simulink model "Lin_test_dsim_quant"  (R2012b)
settings: Solver=FixedStepDiscrete  SolverMode=SingleTasking  StartTime=0.0  StopTime=4096*15  RelTol=1e-3
undefined symbols (not defined in the file or in its folder): fft_stages
libraries: xbsIndex_r4 x7736, casper_library_misc x13, casper_library_sources x12, xps_library x1
(part 33 of 60)

== system Lin_test_dsim_quant/wng0/bus_mult ==
  a : Inport
  b : Inport  Port=2
  a*b_bussify : Subsystem  AncestorBlock=casper_library_flow_control/bus_create  mask(bus_create){inputNum=8}
      mask prompts: inputNum "Number of inputs:"
      mask init:
      | bus_create_init(gcb,...
      |     'inputNum', inputNum);
  a_debus : Subsystem  AncestorBlock=casper_library_flow_control/bus_expand  mask(bus_expand){mode=divisions of arbitrary size, outputNum=1, outputWidth=[21 21 21 21 21 21 21 21], outputBinaryPt=[18 18 18 18 18 18 18 18], outputArithmeticType=[1 1 1 1 1 1 1 1], show_format=on, outputToWorkspace=off, variablePrefix=, outputToModelAsWell=on}
      mask prompts: outputNum "Number of outputs:"; outputWidth "Output width [msb ... lsb]:"; outputBinaryPt "Output binary point position [msb ... lsb]:"; outputArithmeticType "Output arithmetic type (ufix=0, fix=1, bool=2) [msb ... lsb]:"; show_format "Print format string?"; outputToWorkspace "Output to workspace?"; variablePrefix "Variable name prefix:"; outputToModelAsWell "Output to model as well?"
      mask help:
      | Expands a 'bus' made using a bus_create or Xilinx
      | concat block.
      | The input will be divided into the specified number
      | of outputs with the specified arithmetic types.
      | Divisions are made from most significant bit.
      mask init: same as Lin_test_dsim_quant/bus_expand1
      settings: AttributesFormatString=8 outputs: f21.18,f21.18,f21.18,f21.18,f21.18,f21.18,f21.18,f21.18,
      mask TypeOptions mode: divisions of equal size | divisions of arbitrary size
      mask Callback mode: bus_expand_callback();
      mask Callback outputWidth: bus_expand_callback();
      mask Callback outputToWorkspace: bus_expand_callback();
  b_debus : Subsystem  AncestorBlock=casper_library_flow_control/bus_expand  mask(bus_expand){mode=divisions of arbitrary size, outputNum=1, outputWidth=[16 16 16 16 16 16 16 16], outputBinaryPt=[15 15 15 15 15 15 15 15], outputArithmeticType=[0 0 0 0 0 0 0 0], show_format=on, outputToWorkspace=off, variablePrefix=, outputToModelAsWell=on}
      mask prompts: outputNum "Number of outputs:"; outputWidth "Output width [msb ... lsb]:"; outputBinaryPt "Output binary point position [msb ... lsb]:"; outputArithmeticType "Output arithmetic type (ufix=0, fix=1, bool=2) [msb ... lsb]:"; show_format "Print format string?"; outputToWorkspace "Output to workspace?"; variablePrefix "Variable name prefix:"; outputToModelAsWell "Output to model as well?"
      mask help:
      | Expands a 'bus' made using a bus_create or Xilinx
      | concat block.
      | The input will be divided into the specified number
      | of outputs with the specified arithmetic types.
      | Divisions are made from most significant bit.
      mask init: same as Lin_test_dsim_quant/bus_expand1
      settings: AttributesFormatString=8 outputs: uf16.15,uf16.15,uf16.15,uf16.15,uf16.15,uf16.15,uf16.15,uf16.15,
      mask TypeOptions mode: divisions of equal size | divisions of arbitrary size
      mask Callback mode: bus_expand_callback();
      mask Callback outputWidth: bus_expand_callback();
      mask Callback outputToWorkspace: bus_expand_callback();
  mult{1..8} (8 alike) : xbsIndex_r4/Mult  precision=User Defined  arith_type="Signed  (2's comp)"  n_bits=37  bin_pt=33  quantization="Round  (unbiased: +/- Inf)"  overflow=Saturate  en=off  latency=mult_latency  dbl_ovrd=off  use_behavioral_HDL=on  opt=Speed  use_embedded=off  optimum_pipeline=off  pipeline=on  use_rpm=on  placement_style=Triangular  block_type=mult
  repa : Subsystem  AncestorBlock=casper_library_bus/bus_replicate  mask(bus_replicate){replication=1, latency=3, misc=off, implementation=core}
      mask prompts: replication "replication factor"; misc "misc support"; implementation "delay implementation"
      mask help: Output bus formed by replicating input bus a number of times
      mask init:
      | bus_replicate_init(gcb, ...
      |     'replication', replication, ...
      |     'latency', latency, ...
      |     'implementation', implementation, ...
      |     'misc', misc);
      mask TypeOptions implementation: core | behavioral
  repb : Subsystem  AncestorBlock=casper_library_bus/bus_replicate  mask(bus_replicate){replication=8, latency=3, misc=off, implementation=core}
      mask prompts: replication "replication factor"; misc "misc support"; implementation "delay implementation"
      mask help: Output bus formed by replicating input bus a number of times
      mask init:
      | bus_replicate_init(gcb, ...
      |     'replication', replication, ...
      |     'latency', latency, ...
      |     'implementation', implementation, ...
      |     'misc', misc);
      mask TypeOptions implementation: core | behavioral
  a*b : Outport
  wires:
  a/1 -> repa/1(in)
  b/1 -> repb/1(in)
  repa/1(out) -> a_debus/1(bus_in)
  repb/1(out) -> b_debus/1(bus_in)
  a_debus/1(msb_out8) -> mult1/1
  b_debus/1(msb_out8) -> mult1/2
  a_debus/2(out7) -> mult2/1
  b_debus/2(out7) -> mult2/2
  a_debus/3(out6) -> mult3/1
  b_debus/3(out6) -> mult3/2
  a_debus/4(out5) -> mult4/1
  b_debus/4(out5) -> mult4/2
  a_debus/5(out4) -> mult5/1
  b_debus/5(out4) -> mult5/2
  a_debus/6(out3) -> mult6/1
  b_debus/6(out3) -> mult6/2
  a_debus/7(out2) -> mult7/1
  b_debus/7(out2) -> mult7/2
  a_debus/8(lsb_out1) -> mult8/1
  b_debus/8(lsb_out1) -> mult8/2
  mult1/1 -> a*b_bussify/1(in1)
  mult2/1 -> a*b_bussify/2(in2)
  mult3/1 -> a*b_bussify/3(in3)
  mult4/1 -> a*b_bussify/4(in4)
  mult5/1 -> a*b_bussify/5(in5)
  mult6/1 -> a*b_bussify/6(in6)
  mult7/1 -> a*b_bussify/7(in7)
  mult8/1 -> a*b_bussify/8(in8)
  a*b_bussify/1(bus_out) -> a*b/1

== system Lin_test_dsim_quant/wng0/pipeline2 ==
  d : Inport
  Register0 : xbsIndex_r4/Register  init=0  rst=off  en=off  dbl_ovrd=off  block_type=register
      settings: block_version=11.4
  Register1 : xbsIndex_r4/Register  init=0  rst=off  en=off  dbl_ovrd=off  block_type=register
      settings: block_version=11.4
  q : Outport
  wires:
  Register0/1 -> Register1/1
  d/1 -> Register0/1
  Register1/1 -> q/1

== system Lin_test_dsim_quant/wng0/pipeline3 ==
  d : Inport
  Register0 : xbsIndex_r4/Register  init=0  rst=off  en=off  dbl_ovrd=off  block_type=register
      settings: block_version=11.4
  Register1 : xbsIndex_r4/Register  init=0  rst=off  en=off  dbl_ovrd=off  block_type=register
      settings: block_version=11.4
  q : Outport
  wires:
  Register1/1 -> q/1
  d/1 -> Register0/1
  Register0/1 -> Register1/1

== system Lin_test_dsim_quant/wng0/pipeline4 ==
  d : Inport
  Register0 : xbsIndex_r4/Register  init=0  rst=off  en=off  dbl_ovrd=off  block_type=register
      settings: block_version=11.4
  Register1 : xbsIndex_r4/Register  init=0  rst=off  en=off  dbl_ovrd=off  block_type=register
      settings: block_version=11.4
  q : Outport
  wires:
  Register0/1 -> Register1/1
  d/1 -> Register0/1
  Register1/1 -> q/1

== system Lin_test_dsim_quant/wng0/pipeline41 ==
  d : Inport
  Register0 : xbsIndex_r4/Register  init=0  rst=off  en=off  dbl_ovrd=off  block_type=register
      settings: block_version=11.4
  Register1 : xbsIndex_r4/Register  init=0  rst=off  en=off  dbl_ovrd=off  block_type=register
      settings: block_version=11.4
  q : Outport
  wires:
  Register0/1 -> Register1/1
  d/1 -> Register0/1
  Register1/1 -> q/1

== system Lin_test_dsim_quant/wng0/pipeline5 ==
  d : Inport
  Register0 : xbsIndex_r4/Register  init=0  rst=off  en=off  dbl_ovrd=off  block_type=register
      settings: block_version=11.4
  Register1 : xbsIndex_r4/Register  init=0  rst=off  en=off  dbl_ovrd=off  block_type=register
      settings: block_version=11.4
  q : Outport
  wires:
  Register1/1 -> q/1
  d/1 -> Register0/1
  Register0/1 -> Register1/1

== system Lin_test_dsim_quant/wng0/wgn1 ==
  seed : Inport
  ld : Inport  Port=2
  rst : Inport  Port=3
  tt800_uprng : Subsystem  AncestorBlock=casper_library_sources/tt800_uprng  mask(TT800 Uniform Psedo-Random Number Generator){seed=seed}
      mask help: The TT800 is a high quality pseudo-random number generator based on a "twisted generialized linear feedback shift register". Its output sequence repeats after 2^800 samples (~10^240 samples). For more info see: Matsumoto, M. and Kurita, Y. 1994. "Twisted GFSR generators II", ACM Trans. Model. Comput. Simul. 4, 3 (Jul. 1994), 254-266 (http://doi.acm.org/10.1145/189443.189445).
      mask init:
      | set_param([gcb,'/tt800_seed_gen/LFSR'],'rst_value',sprintf('''%08X''', seed));
      mask Help: Initial seed is specified by a mask parameter at design time.  Can be reseeded at runtime by applying a UFix_32_0 value on the seed input and pulsing the load port (ld) high for one cycle.  Holding the load port high for more than one cycle is allowed, but it affects the generator in undocumented ways.  Drill down into the subsystem if you want to learn more.
      mask Display:
      | port_label('input',1,'seed');
      | port_label('input',2,'ld');
      | port_label('output',1,'u');
  u2n : casper_library_sources/u2n  hideme=off
      link override SineCosine: partspresent=SIN_COS_LUT_only  dds_clock_rate=100  channels=1  parameter_entry=Hardware_Parameters  spurious_free_dynamic_range=36  frequency_resolution=0.4  noise_shaping=None  phase_width=11  output_width=10  output_selection=Sine_and_Cosine  negative_sine=off  negative_cosine=off  amplitude_mode=Full_Range  memory_type=Block_ROM  optimization_goal=Auto  dsp48_use=Minimal  latency_configuration=Auto  latency=6  has_phase_out=off  sclr_pin=off  clock_enable=off  rfd=off  rdy=off  channel_pin=off  explicit_period=off  period=1  phase_increment=Fixed  output_frequency1=0  output_frequency2=0  output_frequency3=0  output_frequency4=0  output_frequency5=0  output_frequency6=0  output_frequency7=0  output_frequency8=0  output_frequency9=0  output_frequency10=0  output_frequency11=0  output_frequency12=0  output_frequency13=0  output_frequency14=0  output_frequency15=0  output_frequency16=0  pinc1='0'  pinc2='0'  pinc3='0'  pinc4='0'  pinc5='0'  pinc6='0'  pinc7='0'  pinc8='0'  pinc9='0'  pinc10='0'  pinc11='0'  pinc12='0'  pinc13='0'  pinc14='0'  pinc15='0'  pinc16='0'  phase_offset=None  phase_offset_angles1=0  phase_offset_angles2=0  phase_offset_angles3=0  phase_offset_angles4=0  phase_offset_angles5=0  phase_offset_angles6=0  phase_offset_angles7=0  phase_offset_angles8=0  phase_offset_angles9=0  phase_offset_angles10=0  phase_offset_angles11=0  phase_offset_angles12=0  phase_offset_angles13=0  phase_offset_angles14=0  phase_offset_angles15=0  phase_offset_angles16=0  poff1='0'  poff2='0'  poff3='0'  poff4='0'  poff5='0'  poff6='0'  poff7='0'  poff8='0'  poff9='0'  poff10='0'  poff11='0'  poff12='0'  poff13='0'  poff14='0'  poff15='0'  poff16='0'  por_mode=false  gui_behaviour=Sysgen  ip_name=DDS Compiler  ip_version=4.0  dsptool_ready=true  wrapper_available=true  port_translation_map={ 'ce' => 'en', 'sclr' => 'rst' }  ipcore_xco_need_fpga_part=true  ipcore_fpga_part=xlipgetpartsetting(gcb, {'virtex4', 'xc4vsx35', '-10', 'ff668'})  ipcore_usecache=true  ipcore_useipmodelcache=true  ipcore_verbose=false
      link override log_lut: depth=2^11  initVector=sqrt(-2*log(linspace(2^-11,1,2^11)))  distributed_mem=Block RAM  rst=off  init_reg=0  en=off  latency=6  gui_display_data_type=Fixed-point  arith_type=Unsigned  n_bits=11  bin_pt=9  preci_type=Single  exp_width=8  frac_width=24  dbl_ovrd=off  optimize=Area  use_rpm=off
      link override log_lut: xl_area=[0 0 1 0 0 0 0]
  n1 : Outport
  n2 : Outport  Port=2
  wires:
  u2n/2 -> n2/1
  ld/1 -> tt800_uprng/2(ld)
  u2n/1 -> n1/1
  seed/1 -> tt800_uprng/1(seed)
  tt800_uprng/1(u) -> u2n/1
  rst/1 -> tt800_uprng/3(rst)

== system Lin_test_dsim_quant/wng0/wgn2 ==
  seed : Inport
  ld : Inport  Port=2
  rst : Inport  Port=3
  tt800_uprng : Subsystem  AncestorBlock=casper_library_sources/tt800_uprng  mask(TT800 Uniform Psedo-Random Number Generator){seed=seed}
      mask help: The TT800 is a high quality pseudo-random number generator based on a "twisted generialized linear feedback shift register". Its output sequence repeats after 2^800 samples (~10^240 samples). For more info see: Matsumoto, M. and Kurita, Y. 1994. "Twisted GFSR generators II", ACM Trans. Model. Comput. Simul. 4, 3 (Jul. 1994), 254-266 (http://doi.acm.org/10.1145/189443.189445).
      mask init:
      | set_param([gcb,'/tt800_seed_gen/LFSR'],'rst_value',sprintf('''%08X''', seed));
      mask Help: Initial seed is specified by a mask parameter at design time.  Can be reseeded at runtime by applying a UFix_32_0 value on the seed input and pulsing the load port (ld) high for one cycle.  Holding the load port high for more than one cycle is allowed, but it affects the generator in undocumented ways.  Drill down into the subsystem if you want to learn more.
      mask Display:
      | port_label('input',1,'seed');
      | port_label('input',2,'ld');
      | port_label('output',1,'u');
  u2n : casper_library_sources/u2n  hideme=off
      link override SineCosine: partspresent=SIN_COS_LUT_only  dds_clock_rate=100  channels=1  parameter_entry=Hardware_Parameters  spurious_free_dynamic_range=36  frequency_resolution=0.4  noise_shaping=None  phase_width=11  output_width=10  output_selection=Sine_and_Cosine  negative_sine=off  negative_cosine=off  amplitude_mode=Full_Range  memory_type=Block_ROM  optimization_goal=Auto  dsp48_use=Minimal  latency_configuration=Auto  latency=6  has_phase_out=off  sclr_pin=off  clock_enable=off  rfd=off  rdy=off  channel_pin=off  explicit_period=off  period=1  phase_increment=Fixed  output_frequency1=0  output_frequency2=0  output_frequency3=0  output_frequency4=0  output_frequency5=0  output_frequency6=0  output_frequency7=0  output_frequency8=0  output_frequency9=0  output_frequency10=0  output_frequency11=0  output_frequency12=0  output_frequency13=0  output_frequency14=0  output_frequency15=0  output_frequency16=0  pinc1='0'  pinc2='0'  pinc3='0'  pinc4='0'  pinc5='0'  pinc6='0'  pinc7='0'  pinc8='0'  pinc9='0'  pinc10='0'  pinc11='0'  pinc12='0'  pinc13='0'  pinc14='0'  pinc15='0'  pinc16='0'  phase_offset=None  phase_offset_angles1=0  phase_offset_angles2=0  phase_offset_angles3=0  phase_offset_angles4=0  phase_offset_angles5=0  phase_offset_angles6=0  phase_offset_angles7=0  phase_offset_angles8=0  phase_offset_angles9=0  phase_offset_angles10=0  phase_offset_angles11=0  phase_offset_angles12=0  phase_offset_angles13=0  phase_offset_angles14=0  phase_offset_angles15=0  phase_offset_angles16=0  poff1='0'  poff2='0'  poff3='0'  poff4='0'  poff5='0'  poff6='0'  poff7='0'  poff8='0'  poff9='0'  poff10='0'  poff11='0'  poff12='0'  poff13='0'  poff14='0'  poff15='0'  poff16='0'  por_mode=false  gui_behaviour=Sysgen  ip_name=DDS Compiler  ip_version=4.0  dsptool_ready=true  wrapper_available=true  port_translation_map={ 'ce' => 'en', 'sclr' => 'rst' }  ipcore_xco_need_fpga_part=true  ipcore_fpga_part=xlipgetpartsetting(gcb, {'virtex4', 'xc4vsx35', '-10', 'ff668'})  ipcore_usecache=true  ipcore_useipmodelcache=true  ipcore_verbose=false
      link override log_lut: depth=2^11  initVector=sqrt(-2*log(linspace(2^-11,1,2^11)))  distributed_mem=Block RAM  rst=off  init_reg=0  en=off  latency=6  gui_display_data_type=Fixed-point  arith_type=Unsigned  n_bits=11  bin_pt=9  preci_type=Single  exp_width=8  frac_width=24  dbl_ovrd=off  optimize=Area  use_rpm=off
      link override log_lut: xl_area=[0 0 1 0 0 0 0]
  n1 : Outport
  n2 : Outport  Port=2
  wires:
  u2n/2 -> n2/1
  ld/1 -> tt800_uprng/2(ld)
  u2n/1 -> n1/1
  seed/1 -> tt800_uprng/1(seed)
  tt800_uprng/1(u) -> u2n/1
  rst/1 -> tt800_uprng/3(rst)

== system Lin_test_dsim_quant/wng0/wgn3 ==
  seed : Inport
  ld : Inport  Port=2
  rst : Inport  Port=3
  tt800_uprng : Subsystem  AncestorBlock=casper_library_sources/tt800_uprng  mask(TT800 Uniform Psedo-Random Number Generator){seed=seed}
      mask help: The TT800 is a high quality pseudo-random number generator based on a "twisted generialized linear feedback shift register". Its output sequence repeats after 2^800 samples (~10^240 samples). For more info see: Matsumoto, M. and Kurita, Y. 1994. "Twisted GFSR generators II", ACM Trans. Model. Comput. Simul. 4, 3 (Jul. 1994), 254-266 (http://doi.acm.org/10.1145/189443.189445).
      mask init:
      | set_param([gcb,'/tt800_seed_gen/LFSR'],'rst_value',sprintf('''%08X''', seed));
      mask Help: Initial seed is specified by a mask parameter at design time.  Can be reseeded at runtime by applying a UFix_32_0 value on the seed input and pulsing the load port (ld) high for one cycle.  Holding the load port high for more than one cycle is allowed, but it affects the generator in undocumented ways.  Drill down into the subsystem if you want to learn more.
      mask Display:
      | port_label('input',1,'seed');
      | port_label('input',2,'ld');
      | port_label('output',1,'u');
  u2n : casper_library_sources/u2n  hideme=off
      link override SineCosine: partspresent=SIN_COS_LUT_only  dds_clock_rate=100  channels=1  parameter_entry=Hardware_Parameters  spurious_free_dynamic_range=36  frequency_resolution=0.4  noise_shaping=None  phase_width=11  output_width=10  output_selection=Sine_and_Cosine  negative_sine=off  negative_cosine=off  amplitude_mode=Full_Range  memory_type=Block_ROM  optimization_goal=Auto  dsp48_use=Minimal  latency_configuration=Auto  latency=6  has_phase_out=off  sclr_pin=off  clock_enable=off  rfd=off  rdy=off  channel_pin=off  explicit_period=off  period=1  phase_increment=Fixed  output_frequency1=0  output_frequency2=0  output_frequency3=0  output_frequency4=0  output_frequency5=0  output_frequency6=0  output_frequency7=0  output_frequency8=0  output_frequency9=0  output_frequency10=0  output_frequency11=0  output_frequency12=0  output_frequency13=0  output_frequency14=0  output_frequency15=0  output_frequency16=0  pinc1='0'  pinc2='0'  pinc3='0'  pinc4='0'  pinc5='0'  pinc6='0'  pinc7='0'  pinc8='0'  pinc9='0'  pinc10='0'  pinc11='0'  pinc12='0'  pinc13='0'  pinc14='0'  pinc15='0'  pinc16='0'  phase_offset=None  phase_offset_angles1=0  phase_offset_angles2=0  phase_offset_angles3=0  phase_offset_angles4=0  phase_offset_angles5=0  phase_offset_angles6=0  phase_offset_angles7=0  phase_offset_angles8=0  phase_offset_angles9=0  phase_offset_angles10=0  phase_offset_angles11=0  phase_offset_angles12=0  phase_offset_angles13=0  phase_offset_angles14=0  phase_offset_angles15=0  phase_offset_angles16=0  poff1='0'  poff2='0'  poff3='0'  poff4='0'  poff5='0'  poff6='0'  poff7='0'  poff8='0'  poff9='0'  poff10='0'  poff11='0'  poff12='0'  poff13='0'  poff14='0'  poff15='0'  poff16='0'  por_mode=false  gui_behaviour=Sysgen  ip_name=DDS Compiler  ip_version=4.0  dsptool_ready=true  wrapper_available=true  port_translation_map={ 'ce' => 'en', 'sclr' => 'rst' }  ipcore_xco_need_fpga_part=true  ipcore_fpga_part=xlipgetpartsetting(gcb, {'virtex4', 'xc4vsx35', '-10', 'ff668'})  ipcore_usecache=true  ipcore_useipmodelcache=true  ipcore_verbose=false
      link override log_lut: depth=2^11  initVector=sqrt(-2*log(linspace(2^-11,1,2^11)))  distributed_mem=Block RAM  rst=off  init_reg=0  en=off  latency=6  gui_display_data_type=Fixed-point  arith_type=Unsigned  n_bits=11  bin_pt=9  preci_type=Single  exp_width=8  frac_width=24  dbl_ovrd=off  optimize=Area  use_rpm=off
      link override log_lut: xl_area=[0 0 1 0 0 0 0]
  n1 : Outport
  n2 : Outport  Port=2
  wires:
  u2n/2 -> n2/1
  ld/1 -> tt800_uprng/2(ld)
  u2n/1 -> n1/1
  seed/1 -> tt800_uprng/1(seed)
  tt800_uprng/1(u) -> u2n/1
  rst/1 -> tt800_uprng/3(rst)

== system Lin_test_dsim_quant/wng0/wgn4 ==
  seed : Inport
  ld : Inport  Port=2
  rst : Inport  Port=3
  tt800_uprng : Subsystem  AncestorBlock=casper_library_sources/tt800_uprng  mask(TT800 Uniform Psedo-Random Number Generator){seed=seed}
      mask help: The TT800 is a high quality pseudo-random number generator based on a "twisted generialized linear feedback shift register". Its output sequence repeats after 2^800 samples (~10^240 samples). For more info see: Matsumoto, M. and Kurita, Y. 1994. "Twisted GFSR generators II", ACM Trans. Model. Comput. Simul. 4, 3 (Jul. 1994), 254-266 (http://doi.acm.org/10.1145/189443.189445).
      mask init:
      | set_param([gcb,'/tt800_seed_gen/LFSR'],'rst_value',sprintf('''%08X''', seed));
      mask Help: Initial seed is specified by a mask parameter at design time.  Can be reseeded at runtime by applying a UFix_32_0 value on the seed input and pulsing the load port (ld) high for one cycle.  Holding the load port high for more than one cycle is allowed, but it affects the generator in undocumented ways.  Drill down into the subsystem if you want to learn more.
      mask Display:
      | port_label('input',1,'seed');
      | port_label('input',2,'ld');
      | port_label('output',1,'u');
  u2n : casper_library_sources/u2n  hideme=off
      link override SineCosine: partspresent=SIN_COS_LUT_only  dds_clock_rate=100  channels=1  parameter_entry=Hardware_Parameters  spurious_free_dynamic_range=36  frequency_resolution=0.4  noise_shaping=None  phase_width=11  output_width=10  output_selection=Sine_and_Cosine  negative_sine=off  negative_cosine=off  amplitude_mode=Full_Range  memory_type=Block_ROM  optimization_goal=Auto  dsp48_use=Minimal  latency_configuration=Auto  latency=6  has_phase_out=off  sclr_pin=off  clock_enable=off  rfd=off  rdy=off  channel_pin=off  explicit_period=off  period=1  phase_increment=Fixed  output_frequency1=0  output_frequency2=0  output_frequency3=0  output_frequency4=0  output_frequency5=0  output_frequency6=0  output_frequency7=0  output_frequency8=0  output_frequency9=0  output_frequency10=0  output_frequency11=0  output_frequency12=0  output_frequency13=0  output_frequency14=0  output_frequency15=0  output_frequency16=0  pinc1='0'  pinc2='0'  pinc3='0'  pinc4='0'  pinc5='0'  pinc6='0'  pinc7='0'  pinc8='0'  pinc9='0'  pinc10='0'  pinc11='0'  pinc12='0'  pinc13='0'  pinc14='0'  pinc15='0'  pinc16='0'  phase_offset=None  phase_offset_angles1=0  phase_offset_angles2=0  phase_offset_angles3=0  phase_offset_angles4=0  phase_offset_angles5=0  phase_offset_angles6=0  phase_offset_angles7=0  phase_offset_angles8=0  phase_offset_angles9=0  phase_offset_angles10=0  phase_offset_angles11=0  phase_offset_angles12=0  phase_offset_angles13=0  phase_offset_angles14=0  phase_offset_angles15=0  phase_offset_angles16=0  poff1='0'  poff2='0'  poff3='0'  poff4='0'  poff5='0'  poff6='0'  poff7='0'  poff8='0'  poff9='0'  poff10='0'  poff11='0'  poff12='0'  poff13='0'  poff14='0'  poff15='0'  poff16='0'  por_mode=false  gui_behaviour=Sysgen  ip_name=DDS Compiler  ip_version=4.0  dsptool_ready=true  wrapper_available=true  port_translation_map={ 'ce' => 'en', 'sclr' => 'rst' }  ipcore_xco_need_fpga_part=true  ipcore_fpga_part=xlipgetpartsetting(gcb, {'virtex4', 'xc4vsx35', '-10', 'ff668'})  ipcore_usecache=true  ipcore_useipmodelcache=true  ipcore_verbose=false
      link override log_lut: depth=2^11  initVector=sqrt(-2*log(linspace(2^-11,1,2^11)))  distributed_mem=Block RAM  rst=off  init_reg=0  en=off  latency=6  gui_display_data_type=Fixed-point  arith_type=Unsigned  n_bits=11  bin_pt=9  preci_type=Single  exp_width=8  frac_width=24  dbl_ovrd=off  optimize=Area  use_rpm=off
      link override log_lut: xl_area=[0 0 1 0 0 0 0]
  n1 : Outport
  n2 : Outport  Port=2
  wires:
  u2n/2 -> n2/1
  ld/1 -> tt800_uprng/2(ld)
  u2n/1 -> n1/1
  seed/1 -> tt800_uprng/1(seed)
  tt800_uprng/1(u) -> u2n/1
  rst/1 -> tt800_uprng/3(rst)

== system Lin_test_dsim_quant/wng1/bus_convert ==
  din : Inport
  bussify : Subsystem  AncestorBlock=casper_library_flow_control/bus_create  mask(bus_create){inputNum=8}
      mask prompts: inputNum "Number of inputs:"
      mask init:
      | bus_create_init(gcb,...
      |     'inputNum', inputNum);
  conv1 : Subsystem  AncestorBlock=casper_library_misc/convert  mask(convert){bin_pt_in=33, n_bits_out=20, bin_pt_out=19, quantization=Round  (unbiased: +/- Inf), overflow=Saturate, latency=2}
      mask prompts: bin_pt_in "Binary Point In"; n_bits_out "Bit Width Out"; bin_pt_out "Binary Point Out"
      mask help:
      | Convert input value to the specified bit width and precision.
      |
      | Does not support upscaling number of fractional bits (eg 8_5 to 8_4 is ok, but not 8_4 to 8_5).
      mask init: same as Lin_test_dsim_quant/bus_convert10/conv1
      settings: AttributesFormatString=|
      | N_33 ==> 20_19
      | round inf, saturate
      | latency = 2
      mask Help:
      | <pre>
      | Description::
      | 
      | Outputs converted version of the input.
      | 
      | Mask Parameters::
      | 
      | Binary Point In (bin_pt_in): Specifies the binary point location in the input.
      | 
      | Bit Width Out (n_bits_out): Specifies the width of the output.
      | 
      | Binary Point Out (bin_pt_out): Specifies the binary point location in the output.
      | 
      | Quantization (quantization): Specifies quantization handling.
      | 
      | Overflow (overflow): Specifies overflow handling.
      | 
      | Latency (latency): Specifies the latency of the underlying adder block, which is the overall
      | latency of this block as well.
      | </pre>
      mask TypeOptions quantization: Truncate | Round  (unbiased: +/- Inf) | Round  (unbiased: Even Values) | Round  (unbiased: Zero) | Round  (unbiased: Odd Values) | Round  (biased: Up) | Round  (biased: Down)
      mask TypeOptions overflow: Wrap | Saturate | Error
  conv2 : Subsystem  AncestorBlock=casper_library_misc/convert  mask(convert){bin_pt_in=33, n_bits_out=20, bin_pt_out=19, quantization=Round  (unbiased: +/- Inf), overflow=Saturate, latency=2}
      mask prompts: bin_pt_in "Binary Point In"; n_bits_out "Bit Width Out"; bin_pt_out "Binary Point Out"
      mask help:
      | Convert input value to the specified bit width and precision.
      |
      | Does not support upscaling number of fractional bits (eg 8_5 to 8_4 is ok, but not 8_4 to 8_5).
      mask init: same as Lin_test_dsim_quant/bus_convert10/conv1
      settings: AttributesFormatString=|
      | N_33 ==> 20_19
      | round inf, saturate
      | latency = 2
      mask Help:
      | <pre>
      | Description::
      | 
      | Outputs converted version of the input.
      | 
      | Mask Parameters::
      | 
      | Binary Point In (bin_pt_in): Specifies the binary point location in the input.
      | 
      | Bit Width Out (n_bits_out): Specifies the width of the output.
      | 
      | Binary Point Out (bin_pt_out): Specifies the binary point location in the output.
      | 
      | Quantization (quantization): Specifies quantization handling.
      | 
      | Overflow (overflow): Specifies overflow handling.
      | 
      | Latency (latency): Specifies the latency of the underlying adder block, which is the overall
      | latency of this block as well.
      | </pre>
      mask TypeOptions quantization: Truncate | Round  (unbiased: +/- Inf) | Round  (unbiased: Even Values) | Round  (unbiased: Zero) | Round  (unbiased: Odd Values) | Round  (biased: Up) | Round  (biased: Down)
      mask TypeOptions overflow: Wrap | Saturate | Error
  conv3 : Subsystem  AncestorBlock=casper_library_misc/convert  mask(convert){bin_pt_in=33, n_bits_out=20, bin_pt_out=19, quantization=Round  (unbiased: +/- Inf), overflow=Saturate, latency=2}
      mask prompts: bin_pt_in "Binary Point In"; n_bits_out "Bit Width Out"; bin_pt_out "Binary Point Out"
      mask help:
      | Convert input value to the specified bit width and precision.
      |
      | Does not support upscaling number of fractional bits (eg 8_5 to 8_4 is ok, but not 8_4 to 8_5).
      mask init: same as Lin_test_dsim_quant/bus_convert10/conv1
      settings: AttributesFormatString=|
      | N_33 ==> 20_19
      | round inf, saturate
      | latency = 2
      mask Help:
      | <pre>
      | Description::
      | 
      | Outputs converted version of the input.
      | 
      | Mask Parameters::
      | 
      | Binary Point In (bin_pt_in): Specifies the binary point location in the input.
      | 
      | Bit Width Out (n_bits_out): Specifies the width of the output.
      | 
      | Binary Point Out (bin_pt_out): Specifies the binary point location in the output.
      | 
      | Quantization (quantization): Specifies quantization handling.
      | 
      | Overflow (overflow): Specifies overflow handling.
      | 
      | Latency (latency): Specifies the latency of the underlying adder block, which is the overall
      | latency of this block as well.
      | </pre>
      mask TypeOptions quantization: Truncate | Round  (unbiased: +/- Inf) | Round  (unbiased: Even Values) | Round  (unbiased: Zero) | Round  (unbiased: Odd Values) | Round  (biased: Up) | Round  (biased: Down)
      mask TypeOptions overflow: Wrap | Saturate | Error
  conv4 : Subsystem  AncestorBlock=casper_library_misc/convert  mask(convert){bin_pt_in=33, n_bits_out=20, bin_pt_out=19, quantization=Round  (unbiased: +/- Inf), overflow=Saturate, latency=2}
      mask prompts: bin_pt_in "Binary Point In"; n_bits_out "Bit Width Out"; bin_pt_out "Binary Point Out"
      mask help:
      | Convert input value to the specified bit width and precision.
      |
      | Does not support upscaling number of fractional bits (eg 8_5 to 8_4 is ok, but not 8_4 to 8_5).
      mask init: same as Lin_test_dsim_quant/bus_convert10/conv1
      settings: AttributesFormatString=|
      | N_33 ==> 20_19
      | round inf, saturate
      | latency = 2
      mask Help:
      | <pre>
      | Description::
      | 
      | Outputs converted version of the input.
      | 
      | Mask Parameters::
      | 
      | Binary Point In (bin_pt_in): Specifies the binary point location in the input.
      | 
      | Bit Width Out (n_bits_out): Specifies the width of the output.
      | 
      | Binary Point Out (bin_pt_out): Specifies the binary point location in the output.
      | 
      | Quantization (quantization): Specifies quantization handling.
      | 
      | Overflow (overflow): Specifies overflow handling.
      | 
      | Latency (latency): Specifies the latency of the underlying adder block, which is the overall
      | latency of this block as well.
      | </pre>
      mask TypeOptions quantization: Truncate | Round  (unbiased: +/- Inf) | Round  (unbiased: Even Values) | Round  (unbiased: Zero) | Round  (unbiased: Odd Values) | Round  (biased: Up) | Round  (biased: Down)
      mask TypeOptions overflow: Wrap | Saturate | Error
  conv5 : Subsystem  AncestorBlock=casper_library_misc/convert  mask(convert){bin_pt_in=33, n_bits_out=20, bin_pt_out=19, quantization=Round  (unbiased: +/- Inf), overflow=Saturate, latency=2}
      mask prompts: bin_pt_in "Binary Point In"; n_bits_out "Bit Width Out"; bin_pt_out "Binary Point Out"
      mask help:
      | Convert input value to the specified bit width and precision.
      |
      | Does not support upscaling number of fractional bits (eg 8_5 to 8_4 is ok, but not 8_4 to 8_5).
      mask init: same as Lin_test_dsim_quant/bus_convert10/conv1
      settings: AttributesFormatString=|
      | N_33 ==> 20_19
      | round inf, saturate
      | latency = 2
      mask Help:
      | <pre>
      | Description::
      | 
      | Outputs converted version of the input.
      | 
      | Mask Parameters::
      | 
      | Binary Point In (bin_pt_in): Specifies the binary point location in the input.
      | 
      | Bit Width Out (n_bits_out): Specifies the width of the output.
      | 
      | Binary Point Out (bin_pt_out): Specifies the binary point location in the output.
      | 
      | Quantization (quantization): Specifies quantization handling.
      | 
      | Overflow (overflow): Specifies overflow handling.
      | 
      | Latency (latency): Specifies the latency of the underlying adder block, which is the overall
      | latency of this block as well.
      | </pre>
      mask TypeOptions quantization: Truncate | Round  (unbiased: +/- Inf) | Round  (unbiased: Even Values) | Round  (unbiased: Zero) | Round  (unbiased: Odd Values) | Round  (biased: Up) | Round  (biased: Down)
      mask TypeOptions overflow: Wrap | Saturate | Error
  conv6 : Subsystem  AncestorBlock=casper_library_misc/convert  mask(convert){bin_pt_in=33, n_bits_out=20, bin_pt_out=19, quantization=Round  (unbiased: +/- Inf), overflow=Saturate, latency=2}
      mask prompts: bin_pt_in "Binary Point In"; n_bits_out "Bit Width Out"; bin_pt_out "Binary Point Out"
      mask help:
      | Convert input value to the specified bit width and precision.
      |
      | Does not support upscaling number of fractional bits (eg 8_5 to 8_4 is ok, but not 8_4 to 8_5).
      mask init: same as Lin_test_dsim_quant/bus_convert10/conv1
      settings: AttributesFormatString=|
      | N_33 ==> 20_19
      | round inf, saturate
      | latency = 2
      mask Help:
      | <pre>
      | Description::
      | 
      | Outputs converted version of the input.
      | 
      | Mask Parameters::
      | 
      | Binary Point In (bin_pt_in): Specifies the binary point location in the input.
      | 
      | Bit Width Out (n_bits_out): Specifies the width of the output.
      | 
      | Binary Point Out (bin_pt_out): Specifies the binary point location in the output.
      | 
      | Quantization (quantization): Specifies quantization handling.
      | 
      | Overflow (overflow): Specifies overflow handling.
      | 
      | Latency (latency): Specifies the latency of the underlying adder block, which is the overall
      | latency of this block as well.
      | </pre>
      mask TypeOptions quantization: Truncate | Round  (unbiased: +/- Inf) | Round  (unbiased: Even Values) | Round  (unbiased: Zero) | Round  (unbiased: Odd Values) | Round  (biased: Up) | Round  (biased: Down)
      mask TypeOptions overflow: Wrap | Saturate | Error
  conv7 : Subsystem  AncestorBlock=casper_library_misc/convert  mask(convert){bin_pt_in=33, n_bits_out=20, bin_pt_out=19, quantization=Round  (unbiased: +/- Inf), overflow=Saturate, latency=2}
      mask prompts: bin_pt_in "Binary Point In"; n_bits_out "Bit Width Out"; bin_pt_out "Binary Point Out"
      mask help:
      | Convert input value to the specified bit width and precision.
      |
      | Does not support upscaling number of fractional bits (eg 8_5 to 8_4 is ok, but not 8_4 to 8_5).
      mask init: same as Lin_test_dsim_quant/bus_convert10/conv1
      settings: AttributesFormatString=|
      | N_33 ==> 20_19
      | round inf, saturate
      | latency = 2
      mask Help:
      | <pre>
      | Description::
      | 
      | Outputs converted version of the input.
      | 
      | Mask Parameters::
      | 
      | Binary Point In (bin_pt_in): Specifies the binary point location in the input.
      | 
      | Bit Width Out (n_bits_out): Specifies the width of the output.
      | 
      | Binary Point Out (bin_pt_out): Specifies the binary point location in the output.
      | 
      | Quantization (quantization): Specifies quantization handling.
      | 
      | Overflow (overflow): Specifies overflow handling.
      | 
      | Latency (latency): Specifies the latency of the underlying adder block, which is the overall
      | latency of this block as well.
      | </pre>
      mask TypeOptions quantization: Truncate | Round  (unbiased: +/- Inf) | Round  (unbiased: Even Values) | Round  (unbiased: Zero) | Round  (unbiased: Odd Values) | Round  (biased: Up) | Round  (biased: Down)
      mask TypeOptions overflow: Wrap | Saturate | Error
  conv8 : Subsystem  AncestorBlock=casper_library_misc/convert  mask(convert){bin_pt_in=33, n_bits_out=20, bin_pt_out=19, quantization=Round  (unbiased: +/- Inf), overflow=Saturate, latency=2}
      mask prompts: bin_pt_in "Binary Point In"; n_bits_out "Bit Width Out"; bin_pt_out "Binary Point Out"
      mask help:
      | Convert input value to the specified bit width and precision.
      |
      | Does not support upscaling number of fractional bits (eg 8_5 to 8_4 is ok, but not 8_4 to 8_5).
      mask init: same as Lin_test_dsim_quant/bus_convert10/conv1
      settings: AttributesFormatString=|
      | N_33 ==> 20_19
      | round inf, saturate
      | latency = 2
      mask Help:
      | <pre>
      | Description::
      | 
      | Outputs converted version of the input.
      | 
      | Mask Parameters::
      | 
      | Binary Point In (bin_pt_in): Specifies the binary point location in the input.
      | 
      | Bit Width Out (n_bits_out): Specifies the width of the output.
      | 
      | Binary Point Out (bin_pt_out): Specifies the binary point location in the output.
      | 
      | Quantization (quantization): Specifies quantization handling.
      | 
      | Overflow (overflow): Specifies overflow handling.
      | 
      | Latency (latency): Specifies the latency of the underlying adder block, which is the overall
      | latency of this block as well.
      | </pre>
      mask TypeOptions quantization: Truncate | Round  (unbiased: +/- Inf) | Round  (unbiased: Even Values) | Round  (unbiased: Zero) | Round  (unbiased: Odd Values) | Round  (biased: Up) | Round  (biased: Down)
      mask TypeOptions overflow: Wrap | Saturate | Error
  debus : Subsystem  AncestorBlock=casper_library_flow_control/bus_expand  mask(bus_expand){mode=divisions of arbitrary size, outputNum=1, outputWidth=[37 37 37 37 37 37 37 37], outputBinaryPt=[33 33 33 33 33 33 33 33], outputArithmeticType=[1 1 1 1 1 1 1 1], show_format=on, outputToWorkspace=off, variablePrefix=, outputToModelAsWell=on}
      mask prompts: outputNum "Number of outputs:"; outputWidth "Output width [msb ... lsb]:"; outputBinaryPt "Output binary point position [msb ... lsb]:"; outputArithmeticType "Output arithmetic type (ufix=0, fix=1, bool=2) [msb ... lsb]:"; show_format "Print format string?"; outputToWorkspace "Output to workspace?"; variablePrefix "Variable name prefix:"; outputToModelAsWell "Output to model as well?"
      mask help:
      | Expands a 'bus' made using a bus_create or Xilinx
      | concat block.
      | The input will be divided into the specified number
      | of outputs with the specified arithmetic types.
      | Divisions are made from most significant bit.
      mask init: same as Lin_test_dsim_quant/bus_expand1
      settings: AttributesFormatString=8 outputs: f37.33,f37.33,f37.33,f37.33,f37.33,f37.33,f37.33,f37.33,
      mask TypeOptions mode: divisions of equal size | divisions of arbitrary size
      mask Callback mode: bus_expand_callback();
      mask Callback outputWidth: bus_expand_callback();
      mask Callback outputToWorkspace: bus_expand_callback();
  dout : Outport
  wires:
  din/1 -> debus/1(bus_in)
  debus/1(msb_out8) -> conv1/1(in)
  debus/2(out7) -> conv2/1(in)
  debus/3(out6) -> conv3/1(in)
  debus/4(out5) -> conv4/1(in)
  debus/5(out4) -> conv5/1(in)
  debus/6(out3) -> conv6/1(in)
  debus/7(out2) -> conv7/1(in)
  debus/8(lsb_out1) -> conv8/1(in)
  conv1/1(out) -> bussify/1(in1)
  conv2/1(out) -> bussify/2(in2)
  conv3/1(out) -> bussify/3(in3)
  conv4/1(out) -> bussify/4(in4)
  conv5/1(out) -> bussify/5(in5)
  conv6/1(out) -> bussify/6(in6)
  conv7/1(out) -> bussify/7(in7)
  conv8/1(out) -> bussify/8(in8)
  bussify/1(bus_out) -> dout/1

== system Lin_test_dsim_quant/wng1/bus_create12 ==
  in1 : Inport
  in2 : Inport  Port=2
  in3 : Inport  Port=3
  in4 : Inport  Port=4
  in5 : Inport  Port=5
  in6 : Inport  Port=6
  in7 : Inport  Port=7
  in8 : Inport  Port=8
  concatenate : xbsIndex_r4/Concat  num_inputs=8  dbl_ovrd=off  block_type=concat
  reinterpret{1..8} (8 alike) : xbsIndex_r4/Reinterpret  force_arith_type=on  arith_type=Unsigned  force_bin_pt=on  bin_pt=0  block_type=reinterpret
      reinterpret1 settings: infoedit="Changes signal type without altering the binary representation.   You can changed the signal between signed and unsigned, and relocate the binary point.<br><br>Hardware notes: In hardware this block costs nothing.<br><br>Example:  Suppose the input is 6 bits wide, signed, with 2 fractional bits, and the output is forced to unsigned with 0 fractional bits.  Then an input of -2.0 (1110.00 in binary 2's complement) becomes an output of 56 (111000 in binary)."
      reinterpret2 settings: infoedit="Changes signal type without altering the binary representation.   You can changed the signal between signed and unsigned, and relocate the binary point.<br><br>Hardware notes: In hardware this block costs nothing.<br><br>Example:  Suppose the input is 6 bits wide, signed, with 2 fractional bits, and the output is forced to unsigned with 0 fractional bits.  Then an input of -2.0 (1110.00 in binary 2's complement) becomes an output of 56 (111000 in binary)."
  bus_out : Outport
  wires:
  reinterpret8/1 -> concatenate/8
  in8/1 -> reinterpret8/1
  reinterpret7/1 -> concatenate/7
  in7/1 -> reinterpret7/1
  reinterpret6/1 -> concatenate/6
  in6/1 -> reinterpret6/1
  reinterpret5/1 -> concatenate/5
  in5/1 -> reinterpret5/1
  reinterpret4/1 -> concatenate/4
  in4/1 -> reinterpret4/1
  reinterpret3/1 -> concatenate/3
  in3/1 -> reinterpret3/1
  reinterpret2/1 -> concatenate/2
  in2/1 -> reinterpret2/1
  reinterpret1/1 -> concatenate/1
  in1/1 -> reinterpret1/1
  concatenate/1 -> bus_out/1

== system Lin_test_dsim_quant/wng1/bus_expand ==
  bus_in : Inport
  gatewayOut{1..8} (8 alike) : xbsIndex_r4/Gateway Out  inherit_from_input=off  hdl_port=off  timing_constraint=None  locs_specified=off  LOCs={}  UseAsDAC=off  DACChannel='1'  block_type=gatewayout
  reinterpret{1..8} (8 alike) : xbsIndex_r4/Reinterpret  force_arith_type=on  arith_type="Signed  (2's comp)"  force_bin_pt=on  bin_pt=14  block_type=reinterpret
  slice1 : xbsIndex_r4/Slice  nbits=17  boolean_output=off  mode=Upper Bit Location + Width  bit1=-119  base1=MSB of Input  bit0=0  base0=LSB of Input  dbl_ovrd=off  block_type=slice
  slice2 : xbsIndex_r4/Slice  nbits=17  boolean_output=off  mode=Upper Bit Location + Width  bit1=-102  base1=MSB of Input  bit0=0  base0=LSB of Input  dbl_ovrd=off  block_type=slice
  slice3 : xbsIndex_r4/Slice  nbits=17  boolean_output=off  mode=Upper Bit Location + Width  bit1=-85  base1=MSB of Input  bit0=0  base0=LSB of Input  dbl_ovrd=off  block_type=slice
  slice4 : xbsIndex_r4/Slice  nbits=17  boolean_output=off  mode=Upper Bit Location + Width  bit1=-68  base1=MSB of Input  bit0=0  base0=LSB of Input  dbl_ovrd=off  block_type=slice
  slice5 : xbsIndex_r4/Slice  nbits=17  boolean_output=off  mode=Upper Bit Location + Width  bit1=-51  base1=MSB of Input  bit0=0  base0=LSB of Input  dbl_ovrd=off  block_type=slice
  slice6 : xbsIndex_r4/Slice  nbits=17  boolean_output=off  mode=Upper Bit Location + Width  bit1=-34  base1=MSB of Input  bit0=0  base0=LSB of Input  dbl_ovrd=off  block_type=slice
  slice7 : xbsIndex_r4/Slice  nbits=17  boolean_output=off  mode=Upper Bit Location + Width  bit1=-17  base1=MSB of Input  bit0=0  base0=LSB of Input  dbl_ovrd=off  block_type=slice
  slice8 : xbsIndex_r4/Slice  nbits=17  boolean_output=off  mode=Upper Bit Location + Width  bit1=0  base1=MSB of Input  bit0=0  base0=LSB of Input  dbl_ovrd=off  block_type=slice
  toWorkspace1 : ToWorkspace  VariableName=wng1_raw1_1  SampleTime=-1  SaveFormat=Structure With Time
  toWorkspace2 : ToWorkspace  VariableName=wng1_raw1_2  SampleTime=-1  SaveFormat=Structure With Time
  toWorkspace3 : ToWorkspace  VariableName=wng1_raw1_3  SampleTime=-1  SaveFormat=Structure With Time
  toWorkspace4 : ToWorkspace  VariableName=wng1_raw1_4  SampleTime=-1  SaveFormat=Structure With Time
  toWorkspace5 : ToWorkspace  VariableName=wng1_raw1_5  SampleTime=-1  SaveFormat=Structure With Time
  toWorkspace6 : ToWorkspace  VariableName=wng1_raw1_6  SampleTime=-1  SaveFormat=Structure With Time
  toWorkspace7 : ToWorkspace  VariableName=wng1_raw1_7  SampleTime=-1  SaveFormat=Structure With Time
  toWorkspace8 : ToWorkspace  VariableName=wng1_raw1_8  SampleTime=-1  SaveFormat=Structure With Time
  msb_out8 : Outport
  out7 : Outport  Port=2
  out6 : Outport  Port=3
  out5 : Outport  Port=4
  out4 : Outport  Port=5
  out3 : Outport  Port=6
  out2 : Outport  Port=7
  lsb_out1 : Outport  Port=8
  wires:
  bus_in/1 -> slice8/1, slice7/1, slice6/1, slice5/1, slice4/1, slice3/1, slice2/1, slice1/1
  slice8/1 -> reinterpret8/1
  reinterpret8/1 -> gatewayOut8/1, msb_out8/1
  gatewayOut8/1 -> toWorkspace8/1
  slice7/1 -> reinterpret7/1
  reinterpret7/1 -> gatewayOut7/1, out7/1
  gatewayOut7/1 -> toWorkspace7/1
  slice6/1 -> reinterpret6/1
  reinterpret6/1 -> gatewayOut6/1, out6/1
  gatewayOut6/1 -> toWorkspace6/1
  slice5/1 -> reinterpret5/1
  reinterpret5/1 -> gatewayOut5/1, out5/1
  gatewayOut5/1 -> toWorkspace5/1
  slice4/1 -> reinterpret4/1
  reinterpret4/1 -> gatewayOut4/1, out4/1
  gatewayOut4/1 -> toWorkspace4/1
  slice3/1 -> reinterpret3/1
  reinterpret3/1 -> gatewayOut3/1, out3/1
  gatewayOut3/1 -> toWorkspace3/1
  slice2/1 -> reinterpret2/1
  reinterpret2/1 -> gatewayOut2/1, out2/1
  gatewayOut2/1 -> toWorkspace2/1
  slice1/1 -> reinterpret1/1
  reinterpret1/1 -> gatewayOut1/1, lsb_out1/1
  gatewayOut1/1 -> toWorkspace1/1

== system Lin_test_dsim_quant/wng1/bus_expand1 ==
  bus_in : Inport
  gatewayOut{1..8} (8 alike) : xbsIndex_r4/Gateway Out  inherit_from_input=off  hdl_port=off  timing_constraint=None  locs_specified=off  LOCs={}  UseAsDAC=off  DACChannel='1'  block_type=gatewayout
  reinterpret{1..8} (8 alike) : xbsIndex_r4/Reinterpret  force_arith_type=on  arith_type="Signed  (2's comp)"  force_bin_pt=on  bin_pt=29  block_type=reinterpret
  slice1 : xbsIndex_r4/Slice  nbits=33  boolean_output=off  mode=Upper Bit Location + Width  bit1=-231  base1=MSB of Input  bit0=0  base0=LSB of Input  dbl_ovrd=off  block_type=slice
  slice2 : xbsIndex_r4/Slice  nbits=33  boolean_output=off  mode=Upper Bit Location + Width  bit1=-198  base1=MSB of Input  bit0=0  base0=LSB of Input  dbl_ovrd=off  block_type=slice
  slice3 : xbsIndex_r4/Slice  nbits=33  boolean_output=off  mode=Upper Bit Location + Width  bit1=-165  base1=MSB of Input  bit0=0  base0=LSB of Input  dbl_ovrd=off  block_type=slice
  slice4 : xbsIndex_r4/Slice  nbits=33  boolean_output=off  mode=Upper Bit Location + Width  bit1=-132  base1=MSB of Input  bit0=0  base0=LSB of Input  dbl_ovrd=off  block_type=slice
  slice5 : xbsIndex_r4/Slice  nbits=33  boolean_output=off  mode=Upper Bit Location + Width  bit1=-99  base1=MSB of Input  bit0=0  base0=LSB of Input  dbl_ovrd=off  block_type=slice
  slice6 : xbsIndex_r4/Slice  nbits=33  boolean_output=off  mode=Upper Bit Location + Width  bit1=-66  base1=MSB of Input  bit0=0  base0=LSB of Input  dbl_ovrd=off  block_type=slice
  slice7 : xbsIndex_r4/Slice  nbits=33  boolean_output=off  mode=Upper Bit Location + Width  bit1=-33  base1=MSB of Input  bit0=0  base0=LSB of Input  dbl_ovrd=off  block_type=slice
  slice8 : xbsIndex_r4/Slice  nbits=33  boolean_output=off  mode=Upper Bit Location + Width  bit1=0  base1=MSB of Input  bit0=0  base0=LSB of Input  dbl_ovrd=off  block_type=slice
  toWorkspace1 : ToWorkspace  VariableName=wng1_raw2_1  SampleTime=-1  SaveFormat=Structure With Time
  toWorkspace2 : ToWorkspace  VariableName=wng1_raw2_2  SampleTime=-1  SaveFormat=Structure With Time
  toWorkspace3 : ToWorkspace  VariableName=wng1_raw2_3  SampleTime=-1  SaveFormat=Structure With Time
  toWorkspace4 : ToWorkspace  VariableName=wng1_raw2_4  SampleTime=-1  SaveFormat=Structure With Time
  toWorkspace5 : ToWorkspace  VariableName=wng1_raw2_5  SampleTime=-1  SaveFormat=Structure With Time
  toWorkspace6 : ToWorkspace  VariableName=wng1_raw2_6  SampleTime=-1  SaveFormat=Structure With Time
  toWorkspace7 : ToWorkspace  VariableName=wng1_raw2_7  SampleTime=-1  SaveFormat=Structure With Time
  toWorkspace8 : ToWorkspace  VariableName=wng1_raw2_8  SampleTime=-1  SaveFormat=Structure With Time
  msb_out8 : Outport
  out7 : Outport  Port=2
  out6 : Outport  Port=3
  out5 : Outport  Port=4
  out4 : Outport  Port=5
  out3 : Outport  Port=6
  out2 : Outport  Port=7
  lsb_out1 : Outport  Port=8
  wires:
  bus_in/1 -> slice8/1, slice7/1, slice6/1, slice5/1, slice4/1, slice3/1, slice2/1, slice1/1
  slice8/1 -> reinterpret8/1
  reinterpret8/1 -> gatewayOut8/1, msb_out8/1
  gatewayOut8/1 -> toWorkspace8/1
  slice7/1 -> reinterpret7/1
  reinterpret7/1 -> gatewayOut7/1, out7/1
  gatewayOut7/1 -> toWorkspace7/1
  slice6/1 -> reinterpret6/1
  reinterpret6/1 -> gatewayOut6/1, out6/1
  gatewayOut6/1 -> toWorkspace6/1
  slice5/1 -> reinterpret5/1
  reinterpret5/1 -> gatewayOut5/1, out5/1
  gatewayOut5/1 -> toWorkspace5/1
  slice4/1 -> reinterpret4/1
  reinterpret4/1 -> gatewayOut4/1, out4/1
  gatewayOut4/1 -> toWorkspace4/1
  slice3/1 -> reinterpret3/1
  reinterpret3/1 -> gatewayOut3/1, out3/1
  gatewayOut3/1 -> toWorkspace3/1
  slice2/1 -> reinterpret2/1
  reinterpret2/1 -> gatewayOut2/1, out2/1
  gatewayOut2/1 -> toWorkspace2/1
  slice1/1 -> reinterpret1/1
  reinterpret1/1 -> gatewayOut1/1, lsb_out1/1
  gatewayOut1/1 -> toWorkspace1/1
